simulink model "Angle_from_sensor_compat"  (R2019b)
settings: Solver=FixedStepAuto  StartTime=0.0  StopTime=inf  RelTol=1e-3
libraries: arduinosensorlib x1
settings Model: SILPILModeSetting=veronly  ExtModeTrigDuration=2  Creator=Abdou  LastModifiedBy=Abdou
settings OptimizationCC: EnhancedBackFolding=on  PassReuseOutputArgsAs=Individual arguments  ZeroExternalMemoryAtStartup=off  ZeroInternalMemoryAtStartup=off  MaxStackSize=64  OptimizeBlockOrder=speed  DifferentSizesBufferReuse=on  OptimizationCustomize=off  EfficientTunableParamExpr=on
settings DebuggingCC: ParameterTunabilityLossMsg=error
settings HardwareCC: ProdBitPerInt=16  ProdBitPerPointer=16  ProdBitPerSizeT=16  ProdBitPerPtrDiffT=16  ProdLargestAtomicFloat=None  ProdWordSize=8  ProdHWDeviceType=Atmel->AVR
settings SFSimCC: MATLABDynamicMemAlloc=off
settings RTWCC: SystemTargetFile=ert.tlc  HardwareBoard=Arduino Uno  TLCOptions=-aInlineSetEventsForThisBaseRateFcn=TLC_FALSE -aSuppressMultiTaskScheduler=TLC_FALSE -aRateBasedStepFcn=1  TemplateMakefile=ert_default_tmf  Toolchain=Arduino AVR
settings CodeAppCC: ForceParamTrailComments=on  IgnoreCustomStorageClasses=off  OperatorAnnotations=on  SimulinkDataObjDesc=on  SFDataObjDesc=on  InsertBlockDesc=on
settings ERTTargetCC: SupportContinuousTime=on  SupportVariableSizeSignals=on  ExtMode=on  ExtModeStaticAllocSize=250  ExtModeMexArgs='127.0.0.1' 0 17725

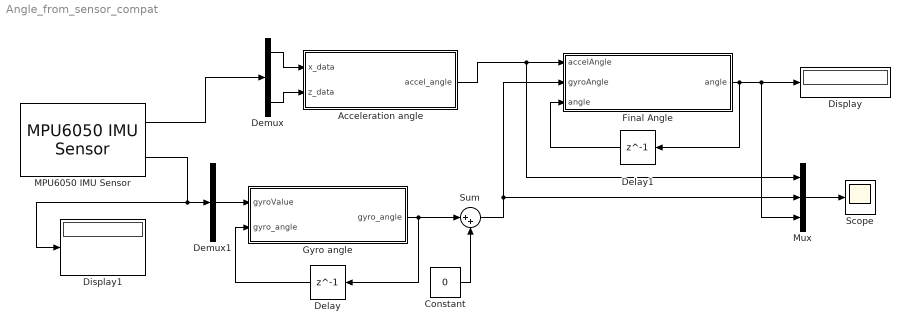
== system Angle_from_sensor_compat ==
  Acceleration angle : MATLAB Function  TreatAsAtomicUnit=on
  Constant : Constant  Value=0
  Delay : Delay  DelayLength=1  InitialCondition=0
  Delay1 : Delay  DelayLength=1  InitialCondition=0
  Demux : Demux  Outputs=3
  Demux1 : Demux  Outputs=3
  Display : Display
  Display1 : Display
  Final Angle : MATLAB Function  TreatAsAtomicUnit=on
  Gyro angle : MATLAB Function  TreatAsAtomicUnit=on
  MPU6050 IMU Sensor : arduinosensorlib/MPU6050 IMU Sensor  SlaveAddress=0x68  Accel=on  AngularRate=on  Temperature=off  Status=off  EulerAngles=off  Quat=off  AccelRange=2G  GyroRange=250 dps  DmpOdr=200 Hz  Dlpf=Accelerometer: 184Hz, Gyroscope: 188Hz  SampleTime=1/100
      settings: SourceProductBaseCode=ARDUINO
  Mux : Mux  Inputs=3
  Scope : Scope
  Sum : Sum  Inputs=|++
  wires:
  MPU6050 IMU Sensor/1 -> Demux/1
  Gyro angle/1(gyro_angle) -> Sum/1, Delay/1
  Delay/1 -> Gyro angle/2("gyro_angle ")
  MPU6050 IMU Sensor/2 -> Display1/1, Demux1/1
  Demux1/2 -> Gyro angle/1(gyroValue)
  Acceleration angle/1(accel_angle) -> Final Angle/1(accelAngle), Mux/1
  Final Angle/1(angle) -> Delay1/1, Mux/3, Display/1
  Delay1/1 -> Final Angle/3("angle ")
  Demux/1 -> Acceleration angle/1(x_data)
  Demux/3 -> Acceleration angle/2(z_data)
  Mux/1 -> Scope/1
  Sum/1 -> Mux/2, Final Angle/2(gyroAngle)
  Constant/1 -> Sum/2

== matlab function Angle_from_sensor_compat/Final Angle ==
  data: accelAngle input; gyroAngle input; angle output; angle input
function angle = Complimentary_filter(accelAngle,gyroAngle,angle)
    filter_coef = 0.98;
    angle = filter_coef * (angle + gyroAngle / 100 ) + (1 - filter_coef) * accelAngle;

== matlab function Angle_from_sensor_compat/Gyro angle ==
  data: gyroValue input; gyro_angle output; gyro_angle input
function gyro_angle = Gyro_angle(gyroValue,gyro_angle)
    offset = 7;
    sensitivity = 1;
    gyroRate = (gyroValue - offset) * sensitivity;
    gyro_angle = gyro_angle - gyroRate / 100.0;

== matlab function Angle_from_sensor_compat/Acceleration angle ==
  data: x_data input; z_data input; accel_angle output
function accel_angle = Accel_angle(x_data,z_data)
    accel_angle = atan2(x_data,z_data) * 180/pi ;
